simulink model "dynamics_track"  (R2021b)
settings: Solver=VariableStepAuto  StartTime=0.0  StopTime=120  RelTol=1e-10  AbsTol=1e-14
values from neighbouring files (symbols this model uses):
  q0 = [-0.8;0;pi]    [SIM01.m]    (also in SIM02.m = [j 0 the(k)]'; SIM03.m = [-1;0;-pi/2]; SIM04.m = [1 1 k]'; SIM05.m = [2;1;2])
  V0 = [0;0]    [SIM06.m]    (also in SIM07.m)
settings Model: Creator=PC  LastModifiedBy=PC
settings DataIOCC: SaveFormat=Array

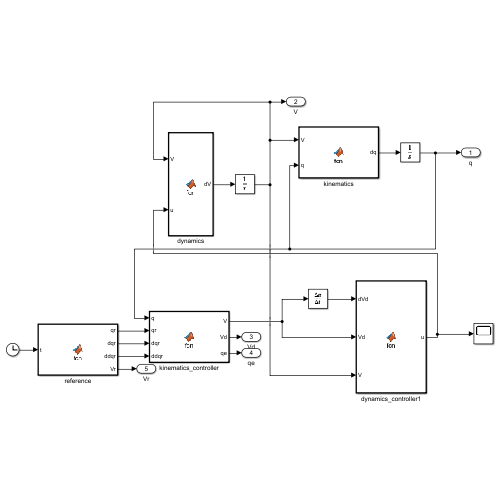
[thumbnail: Simulink's stored preview of the top-level diagram]
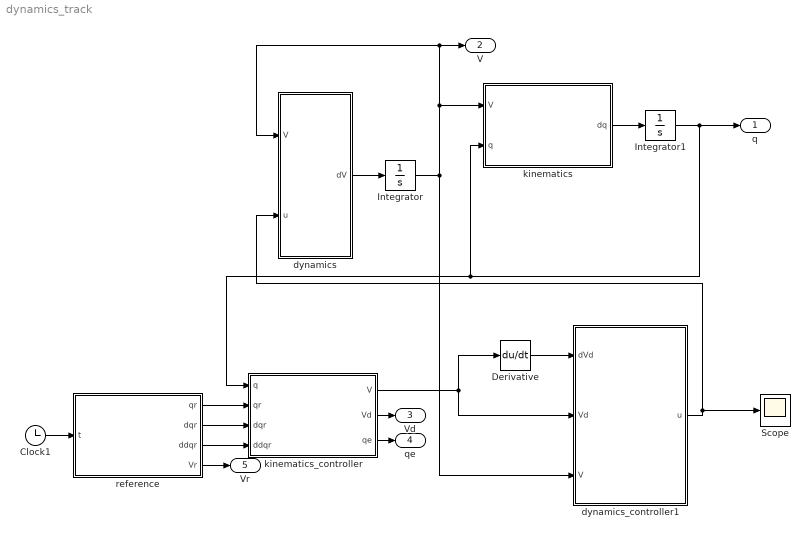
== system dynamics_track ==
  Clock1 : Clock
  Derivative : Derivative
  Integrator : Integrator  InitialCondition=V0
  Integrator1 : Integrator  InitialCondition=q0
  Scope : Scope
  dynamics : MATLAB Function  TreatAsAtomicUnit=on
  dynamics_controller1 : MATLAB Function  TreatAsAtomicUnit=on
  kinematics : MATLAB Function  TreatAsAtomicUnit=on
  kinematics_controller : MATLAB Function  TreatAsAtomicUnit=on
  reference : MATLAB Function  TreatAsAtomicUnit=on
  q : Outport
  V : Outport  Port=2
  Vd : Outport  Port=3
  qe : Outport  Port=4
  Vr : Outport  Port=5
  wires:
  dynamics/1(dV) -> Integrator/1
  Integrator/1 -> dynamics_controller1/3(V), kinematics/1(V), V/1, dynamics/1(V)
  kinematics_controller/1(V) -> dynamics_controller1/2(Vd), Derivative/1
  Derivative/1 -> dynamics_controller1/1(dVd)
  Integrator1/1 -> q/1, kinematics_controller/1(q), kinematics/2(q)
  dynamics_controller1/1(u) -> Scope/1, dynamics/2(u)
  kinematics/1(dq) -> Integrator1/1
  reference/1(qr) -> kinematics_controller/2(qr)
  kinematics_controller/3(qe) -> qe/1
  reference/4(Vr) -> Vr/1
  reference/2(dqr) -> kinematics_controller/3(dqr)
  Clock1/1 -> reference/1(t)
  reference/3(ddqr) -> kinematics_controller/4(ddqr)
  kinematics_controller/2(Vd) -> Vd/1

== matlab function dynamics_track/dynamics ==
  data: V input size=2*1; u input size=2*1; dV output size=2*1
function dV = fcn(V,u)
m=3;
p=0.1;
J=1;
d=0.05;
r=0.05;
L=0.1;
al=m+p;
be=m*d^2+p*L^2+J;
ga=m*d;
M=diag([al,be]);
dV = M^-1*(ga*V(2)*[V(2);-V(1)]+[1 1;L -L]*u/r);

== matlab function dynamics_track/kinematics ==
  data: V input size=2*1; dq output size=3*1; q input size=3*1
function dq = fcn(V,q)
dq=[ cos(q(3))  0
     sin(q(3))  0
      0         1]*V;

== matlab function dynamics_track/kinematics_controller ==
  data: q input size=3*1; V output size=2*1; qr input size=2*1; Vd output size=2*1; dqr input size=2*1; ddqr input size=2*1; qe output size=2*1
function [V,Vd,qe]= fcn(q,qr,dqr,ddqr)
the=atan2(sin(q(3)),cos(q(3)));


xr=qr(1);yr=qr(2);
dxr=dqr(1);dyr=dqr(2);
ddxr=ddqr(1);ddyr=ddqr(2);

k1=0.3;k2=0.3;
vm=0.14;wm=0.24;

al=atan2(dyr+k1*(yr-q(2)),dxr+k1*(xr-q(1)));    
thee=atan2(sin(al-the),cos(al-the));

vp=sqrt((dyr+k1*(yr-q(2)))^2+(dxr+k1*(xr-q(1)))^2);
vd=vp*cos(thee*0.5)^2;
v=min(vd,vm);
dal=((ddyr+k1*dyr-k1*v*sin(the))*cos(al)-(ddxr+k1*dxr-k1*v*cos(the))*sin(al))/((dxr+k1*(xr-q(1)))*cos(al)+(dyr+k1*(yr-q(2)))*sin(al));
wd=dal+2*k2*sin(thee*0.5);
w=sign(wd)*min(abs(wd),wm);
V=[v;w];
Vd=[vd;wd];
qe=q(1:2)-qr;

== matlab function dynamics_track/dynamics_controller1 ==
  data: dVd input size=2*1; u output size=2*1; Vd input size=2*1; V input size=2*1
function u= fcn(dVd,Vd,V)
K=5;
m=3;
p=0.1;
J=1;
d=0.05;
r=0.05;
L=0.1;
al=m+p;
be=m*d^2+p*L^2+J;
ga=m*d;
M=diag([al,be]);
dV=dVd-K*(V-Vd);
C=[1 1;L -L]/r;
u=C^-1*(M*dV-ga*V(2)*[V(2);-V(1)]);

== matlab function dynamics_track/reference ==
  data: qr output size=2*1; dqr output size=2*1; ddqr output size=2*1; Vr output size=2*1; t input
function [qr,dqr,ddqr,Vr]= fcn(t)
da1=0.08;da2=0.04;r=1.5;
qr=[r*sin(da1*t);r*sin(da2*t)];
dqr=[r*da1*cos(da1*t);r*da2*cos(da2*t)];
ddqr=[-r*da1^2*sin(da1*t);-r*da2^2*sin(da2*t)];
ther=atan2(dqr(2),dqr(1));
vr=sqrt(dqr'*dqr);
wr=-[sin(ther) -cos(ther)]*ddqr/vr;
Vr=[vr;wr];
